simulink model "communication_system_latest"  (R2020b)
settings: Solver=VariableStepAuto  StartTime=0.0  StopTime=0.01  RelTol=1e-3
undefined symbols (not defined in the file): magnitude
libraries: commfilt2 x4, commsrccod2 x2, commdigbbndpm3 x2, commblkcod2 x2, dspmathops x2, phaseddetectlib x2, dspsrcs4 x1, commrandsrc3 x1, commsink2 x1, dspvision x1, commchan3 x1
settings Model: Creator=huawei  LastModifiedBy=69553
settings DataIOCC: ReturnWorkspaceOutputs=off

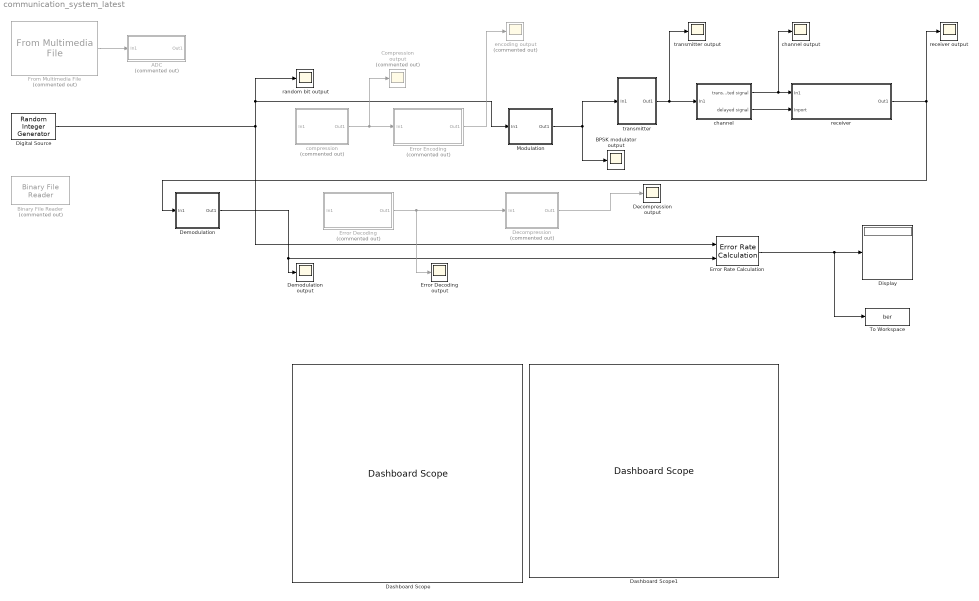
== system communication_system_latest ==
  ADC : Subsystem  Commented=on
  BPSK modulator output : Scope
  Binary File Reader : dspsrcs4/Binary File Reader  Commented=on  Filename=Untitled.bin  HeaderStructure=struct([])  DataType=double  SamplesPerFrame=1024  IsDataComplex=off  NumChannels=1  OutputEOF=off  SampleTime=1  SimulateUsing=Code generation
      settings: SourceProductBaseCode=DS
  Compression output : Scope  Commented=on
  Dashboard Scope : DashboardScope
  Dashboard Scope1 : DashboardScope
  Decompression : Subsystem  Commented=on
  Decompression output : Scope
  Demodulation : Subsystem
  Demodulation output : Scope
  Digital Source : commrandsrc3/Random Integer Generator  SetSize=2  SeedSource=Auto  Seed=0  SampleTime=(1e-4)  SamplesPerFrame=1  OutputDataType=double  SimulateUsing=Interpreted execution
  Display : Display
  Error Decoding : Subsystem  Commented=on
  Error Decoding output : Scope
  Error Encoding : Subsystem  Commented=on
  Error Rate Calculation : commsink2/Error Rate Calculation  N=0  st_delay=0  cp_mode=Entire frame  subframe=[]  PMode=Port  WsName=ErrorVec  RsMode2=off  stop=on  numErr=1000  maxBits=10000
      settings: SourceProductName=Communications Toolbox
  From Multimedia File : dspvision/From Multimedia File  Commented=on  inputFilename=C:\Users\69553\Desktop\UBC\ELEC291\Project 1\project2_audio.wav  readRange=[1 Inf]  loop=on  numPlays=inf  outputStreams=Audio only  videoDataType=single  audioDataType=double  inheritSampleTime=on  userDefinedSampleTime=1/30  noAudioOutput=off  isIntensityVideo=off  fourcc=RGB  colorVideoFormat=Separate color signals  outputEOF=off  dataOrg=Column-major  audioFrameSize=1  computeAudioFrameSize=off  outSamplingMode=Sample based
  Modulation : Subsystem
  To Workspace : ToWorkspace  VariableName=ber  SampleTime=-1
      settings: MaxDataPoints=2  Save2DSignal=2-D array (concatenate along first dimension)
  channel : Subsystem
  channel output : Scope
  compression : Subsystem  Commented=on
  encoding output : Scope  Commented=on
  random bit output : Scope
  receiver : Subsystem
  receiver output : Scope
  transmitter : Subsystem
  transmitter output : Scope
  wires:
  Error Rate Calculation/1 -> To Workspace/1, Display/1
  receiver/1(Out1) -> Demodulation/1(In1), receiver output/1
  Digital Source/1 -> Modulation/1(In1), random bit output/1, Error Rate Calculation/1
  channel/1(transmitted signal) -> receiver/1(In1), channel output/1
  Modulation/1(Out1) -> BPSK modulator output/1, transmitter/1(In1)
  Error Encoding/1(Out1) -> encoding output/1
  compression/1(Out1) -> Error Encoding/1(In1), Compression output/1
  Demodulation/1(Out1) -> Error Rate Calculation/2, Demodulation output/1
  Error Decoding/1(Out1) -> Decompression/1(In1), Error Decoding output/1
  Decompression/1(Out1) -> Decompression output/1
  From Multimedia File/1 -> ADC/1(In1)
  channel/2(delayed signal) -> receiver/2(Inport)
  transmitter/1(Out1) -> transmitter output/1, channel/1(In1)

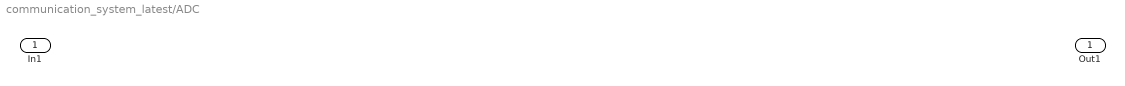
== system communication_system_latest/ADC ==
  In1 : Inport
  Out1 : Outport

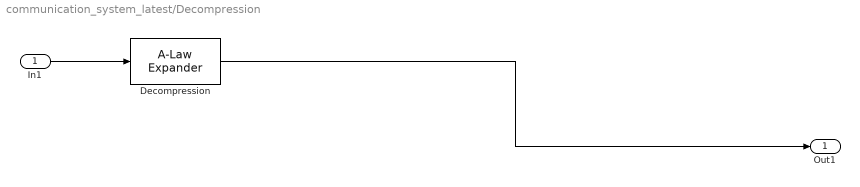
== system communication_system_latest/Decompression ==
  In1 : Inport
  Decompression : commsrccod2/A-Law Expander  A=87.6  V=1
      settings: SourceProductBaseCode=CM
  Out1 : Outport
  wires:
  Decompression/1 -> Out1/1
  In1/1 -> Decompression/1

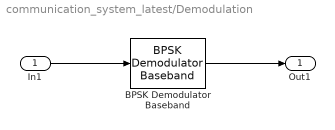
== system communication_system_latest/Demodulation ==
  In1 : Inport
  BPSK Demodulator Baseband : commdigbbndpm3/BPSK Demodulator Baseband  DecType=Hard decision  VarSource=Dialog  Variance=1  Ph=0  outDtype=Inherit via internal rule  derotateFactorWordLen=16  derotateFactorDataTypeStr=Inherit: Same word length as input  derotateFactorLastDataTypeStr=Inherit: Same word length as input
      settings: SourceProductName=Communications Toolbox
  Out1 : Outport
  wires:
  In1/1 -> BPSK Demodulator Baseband/1
  BPSK Demodulator Baseband/1 -> Out1/1

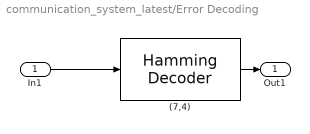
== system communication_system_latest/Error Decoding ==
  In1 : Inport
  (7,4) : commblkcod2/Hamming Decoder  n=7  k=4
      settings: SourceProductBaseCode=CM
  Out1 : Outport
  wires:
  (7,4)/1 -> Out1/1
  In1/1 -> (7,4)/1

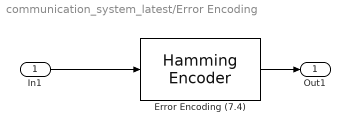
== system communication_system_latest/Error Encoding ==
  In1 : Inport
  "Error Encoding (7.4) " : commblkcod2/Hamming Encoder  n=7  k=4
      settings: SourceProductBaseCode=CM
  Out1 : Outport
  wires:
  "Error Encoding (7.4) "/1 -> Out1/1
  In1/1 -> "Error Encoding (7.4) "/1

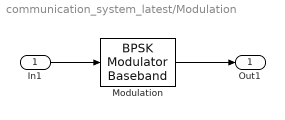
== system communication_system_latest/Modulation ==
  In1 : Inport
  "Modulation " : commdigbbndpm3/BPSK Modulator Baseband  Ph=0  outDtype=double  outWordLen=16  outUDDataType=sfix(16)  outFracLenMode=Best precision  outFracLen=15  outDataTypeStr=double  outLastDataTypeStr=double
  Out1 : Outport
  wires:
  "Modulation "/1 -> Out1/1
  In1/1 -> "Modulation "/1

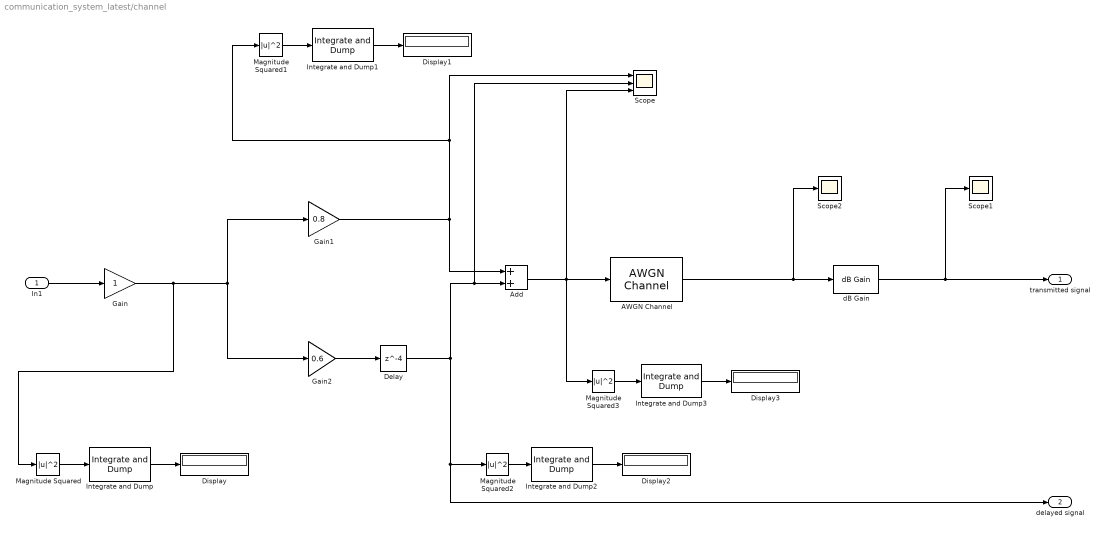
== system communication_system_latest/channel ==
  In1 : Inport
  AWGN Channel : commchan3/AWGN Channel  InputProcessing=Columns as channels (frame based)  seed=67  noiseMode="Signal to noise ratio  (Eb/No)"  EbNodB=12  EsNodB=10  SNRdB=10  bitsPerSym=1  Ps=1  Tsym=1e-4  variance=1
  Add : Sum
  Delay : Delay  DelayLength=4
  Display{,1..3} (4 alike) : Display
  Gain : Gain
  Gain1 : Gain  Gain=0.8
  Gain2 : Gain  Gain=0.6
  Integrate and Dump{,1..3} (4 alike) : commfilt2/Integrate and Dump  obssamples=4  offsetsamples=0  nodump=off  roundingMode=Floor  overflowMode=off  outputDataTypeStr=Inherit: Same as accumulator  outputLastDataTypeStr=Inherit: Same as accumulator
  Magnitude Squared{,1..3} (4 alike) : Math  Operator=magnitude^2  SaturateOnIntegerOverflow=on
  Scope : Scope  NumInputPorts=3
  Scope1 : Scope
  Scope2 : Scope
  dB Gain : dspmathops/dB Gain  dB=-80  intype=Amplitude
      settings: SourceProductBaseCode=DS
  transmitted signal : Outport
  delayed signal : Outport  Port=2
  wires:
  In1/1 -> Gain/1
  Gain/1 -> Magnitude Squared/1, Gain2/1, Gain1/1
  Gain2/1 -> Delay/1
  Magnitude Squared/1 -> Integrate and Dump/1
  Integrate and Dump/1 -> Display/1
  Gain1/1 -> Magnitude Squared1/1, Scope/1, Add/1
  Magnitude Squared1/1 -> Integrate and Dump1/1
  Integrate and Dump1/1 -> Display1/1
  Delay/1 -> delayed signal/1, Magnitude Squared2/1, Scope/2, Add/2
  Magnitude Squared2/1 -> Integrate and Dump2/1
  Integrate and Dump2/1 -> Display2/1
  Add/1 -> Magnitude Squared3/1, AWGN Channel/1, Scope/3
  Magnitude Squared3/1 -> Integrate and Dump3/1
  Integrate and Dump3/1 -> Display3/1
  AWGN Channel/1 -> dB Gain/1, Scope2/1
  dB Gain/1 -> Scope1/1, transmitted signal/1

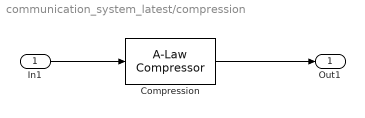
== system communication_system_latest/compression ==
  In1 : Inport
  Compression : commsrccod2/A-Law Compressor  A=87.6  V=1
      settings: SourceProductBaseCode=CM
  Out1 : Outport
  wires:
  In1/1 -> Compression/1
  Compression/1 -> Out1/1

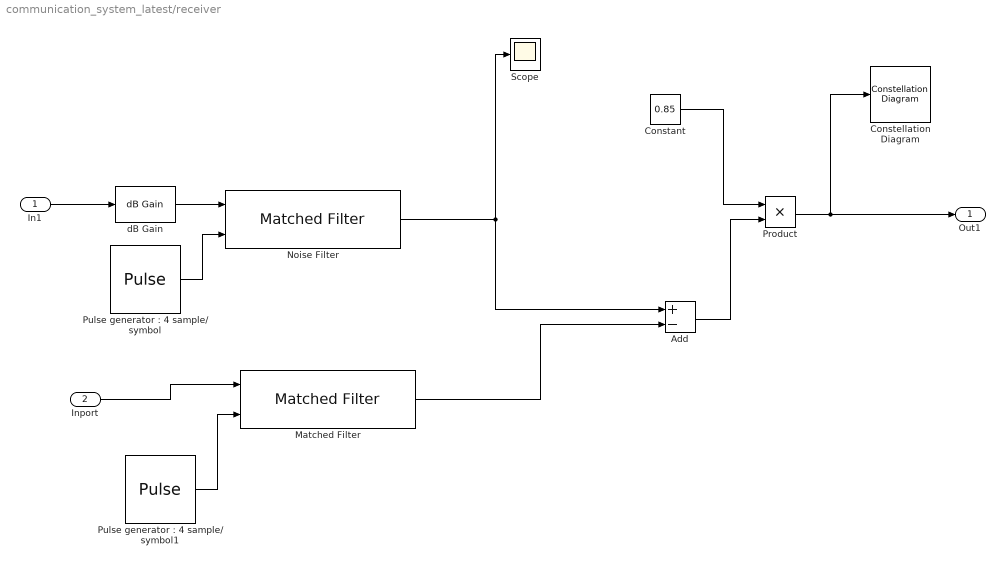
== system communication_system_latest/receiver ==
  In1 : Inport
  Inport : Inport  Port=2
  Add : Sum  Inputs=+-
  Constant : Constant  Value=0.85
  Constellation Diagram : ConstellationDiagram
  Matched Filter : phaseddetectlib/Matched Filter  CoefficientsSource=Input port  Coefficients=[ 1; 1 ]  SpectrumWindow=None  CustomSpectrumWindow=@hamming  SpectrumRange=[ 0, 1e5 ]  SampleRateFromInputCheckbox=on  SampleRate=1e6  SidelobeAttenuation=80  Beta=0.5  Nbar=4  GainOutputPort=off  MaximumNumInputSamplesSource=Auto  MaximumNumInputSamples=100  SimulateUsing=Interpreted execution
      settings: SourceProductBaseCode=AR
  Noise Filter : phaseddetectlib/Matched Filter  CoefficientsSource=Input port  Coefficients=[ 1; 1 ]  SpectrumWindow=None  CustomSpectrumWindow=@hamming  SpectrumRange=[ 0, 1e5 ]  SampleRateFromInputCheckbox=on  SampleRate=1e6  SidelobeAttenuation=80  Beta=0.5  Nbar=4  GainOutputPort=off  MaximumNumInputSamplesSource=Auto  MaximumNumInputSamples=100  SimulateUsing=Interpreted execution
      settings: SourceProductBaseCode=AR
  Product : Product
  "Pulse generator : 4 sample/ symbol" : DiscretePulseGenerator  Period=4  PulseWidth=4  SampleTime=1e-4/4
  "Pulse generator : 4 sample/ symbol1" : DiscretePulseGenerator  Period=4  PulseWidth=4  SampleTime=1e-4/4
  Scope : Scope
  dB Gain : dspmathops/dB Gain  dB=80  intype=Amplitude
      settings: SourceProductBaseCode=DS
  Out1 : Outport
  wires:
  "Pulse generator : 4 sample/ symbol"/1 -> Noise Filter/2
  "Pulse generator : 4 sample/ symbol1"/1 -> Matched Filter/2
  Constant/1 -> Product/1
  Add/1 -> Product/2
  Product/1 -> Out1/1, Constellation Diagram/1
  Inport/1 -> Matched Filter/1
  Matched Filter/1 -> Add/2
  Noise Filter/1 -> Add/1, Scope/1
  In1/1 -> dB Gain/1
  dB Gain/1 -> Noise Filter/1

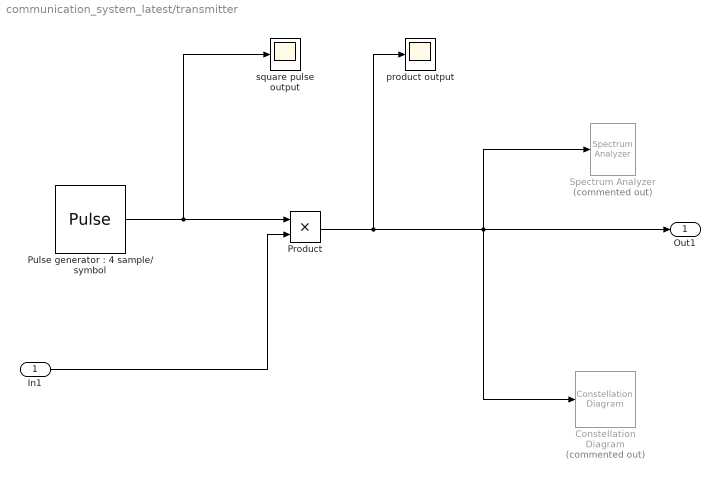
== system communication_system_latest/transmitter ==
  In1 : Inport
  Constellation Diagram : ConstellationDiagram  Commented=on
  Product : Product
  "Pulse generator : 4 sample/ symbol" : DiscretePulseGenerator  Period=4  PulseWidth=4  SampleTime=1e-4/4
  Spectrum Analyzer : SpectrumAnalyzer  Commented=on
  product output : Scope
  square pulse output : Scope
  Out1 : Outport
  wires:
  In1/1 -> Product/2
  Product/1 -> product output/1, Out1/1, Spectrum Analyzer/1, Constellation Diagram/1
  "Pulse generator : 4 sample/ symbol"/1 -> square pulse output/1, Product/1
